simulink library "NullRadarSurveillanceBus"  (R2018b)
settings: Solver=VariableStepAuto  StartTime=0.0  StopTime=10.0  RelTol=1e-3
libraries: signalsLib x1
settings Model: Creator=RA24876  LastModifiedBy=RA24876
settings SFSimCC: SimUseLocalCustomCode=off
settings RTWCC: RTWUseLocalCustomCode=off
settings CodeAppCC: StateflowObjectComments=on

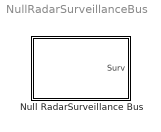
== system NullRadarSurveillanceBus ==
  Null RadarSurveillance Bus : Subsystem  mask(Null RadarSurveillance Bus){}
      mask help: Creates a RadarSurveillance bus signal with all null values. Assign values to elements with a Bus Assignment block.

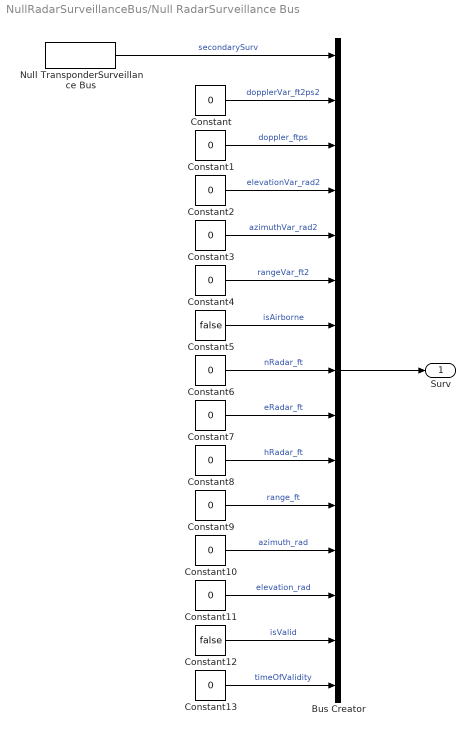
== system NullRadarSurveillanceBus/Null RadarSurveillance Bus ==
  Bus Creator : BusCreator  Inputs='latLonAltEst','timeOfValidity','isValid','enuStateEstimate','covEstimate','newsignal1','newsignal2','newsignal3','newsignal4','newsignal5','newsignal6','newsignal7','newsignal8','newsignal9','newsignal10'  OutDataTypeStr=Bus: RadarSurveillance
  Constant{,1..4,6..11,13} (12 alike) : Constant  Value=0
  Constant12 : Constant  Value=false  OutDataTypeStr=boolean
  Constant5 : Constant  Value=false  OutDataTypeStr=boolean
  Null TransponderSurveillance Bus : signalsLib/Signals/Bus Constructors/Null TransponderSurveillance Bus
      settings: SourceProductName=CASSATTv6: Signals Library
  Surv : Outport  OutDataTypeStr=Bus: RadarSurveillance
  wires:
  Constant13/1 -> Bus Creator/15  "timeOfValidity"
  Constant12/1 -> Bus Creator/14  "isValid"
  Constant11/1 -> Bus Creator/13  "elevation_rad"
  Constant10/1 -> Bus Creator/12  "azimuth_rad"
  Constant9/1 -> Bus Creator/11  "range_ft"
  Constant8/1 -> Bus Creator/10  "hRadar_ft"
  Constant7/1 -> Bus Creator/9  "eRadar_ft"
  Constant6/1 -> Bus Creator/8  "nRadar_ft"
  Constant5/1 -> Bus Creator/7  "isAirborne"
  Constant4/1 -> Bus Creator/6  "rangeVar_ft2"
  Constant3/1 -> Bus Creator/5  "azimuthVar_rad2"
  Constant2/1 -> Bus Creator/4  "elevationVar_rad2"
  Constant1/1 -> Bus Creator/3  "doppler_ftps"
  Constant/1 -> Bus Creator/2  "dopplerVar_ft2ps2"
  Bus Creator/1 -> Surv/1
  Null TransponderSurveillance Bus/1 -> Bus Creator/1  "secondarySurv"
